simulink model "exp2_ModulationDemodulation"  (R2023b)
settings: Solver=VariableStepAuto  StartTime=0.0  StopTime=10.0  RelTol=1e-3
libraries: dspfdesign x1
settings Model: Creator=Student  LastModifiedBy=ketaki mahajan
settings OptimizationCC: ReuseModelBlockBuffer=off

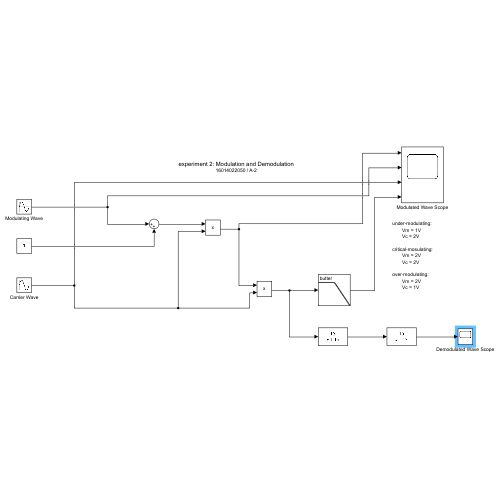
[thumbnail: Simulink's stored preview of the top-level diagram]
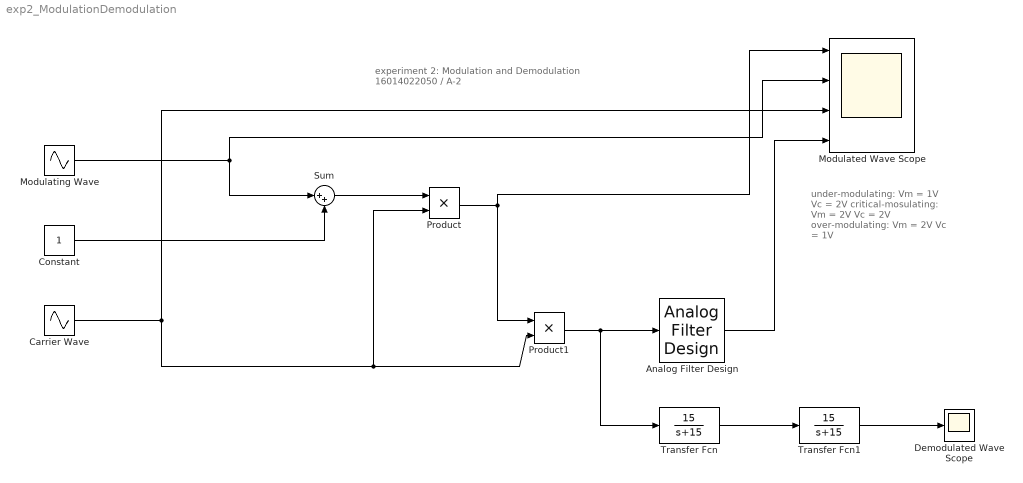
== system exp2_ModulationDemodulation ==
  note: experiment 2: Modulation and Demodulation
      | 16014022050 / A-2
  note: under-modulating:
      | 	Vm = 1V
      | 	Vc = 2V
      |
      | critical-mosulating:
      | 	Vm = 2V
      | 	Vc = 2V
      |
      | over-modulating:
      | 	Vm = 2V
      | 	Vc = 1V
  Analog Filter Design : dspfdesign/Analog Filter Design  method=Butterworth  filttype=Lowpass  N=8  Wlo=30  Whi=80  Rp=2  Rs=40
  Carrier Wave : Sin  Amplitude=2  Frequency=20  SampleTime=0
  Constant : Constant
  Demodulated Wave Scope : Scope
  Modulated Wave Scope : Scope  NumInputPorts=4
  Modulating Wave : Sin  SampleTime=0
  Product : Product
  Product1 : Product
  Sum : Sum  Inputs=|++
  Transfer Fcn : TransferFcn  Numerator=[15]  Denominator=[1 15]
  Transfer Fcn1 : TransferFcn  Numerator=[15]  Denominator=[1 15]
  wires:
  Constant/1 -> Sum/2
  Sum/1 -> Product/1
  Product/1 -> Modulated Wave Scope/1, Product1/1
  Analog Filter Design/1 -> Modulated Wave Scope/4
  Carrier Wave/1 -> Modulated Wave Scope/3, Product/2, Product1/2
  Modulating Wave/1 -> Modulated Wave Scope/2, Sum/1
  Transfer Fcn1/1 -> Demodulated Wave Scope/1
  Product1/1 -> Transfer Fcn/1, Analog Filter Design/1
  Transfer Fcn/1 -> Transfer Fcn1/1
